simulink model "BCS_v1_2018a"  (R2018a)
settings: Solver=ode5  StartTime=0.0  StopTime=inf  FixedStep=sampletime  RelTol=1e-3  EnableMultiTasking=on
values from neighbouring files (symbols this model uses):
  extension_lower = 0    [Ignition.m]
  extension_upper = 1800    [Ignition.m]
  kd4 = 1e-2    (= 0.01)    [Ignition.m]
  kq1 = 0.1    [Ignition.m]
  kq2 = 0.1    [Ignition.m]
  kq3 = 0.1    [Ignition.m]
  lift_lower = 0    [Ignition.m]
  lift_upper = 75    [Ignition.m]
  Max_1 = 5    [Ignition.m]
  Max_2 = 5    [Ignition.m]
  Max_3 = 5    [Ignition.m]
  Max_4 = 10    [Ignition.m]
  Max_rot = 5    [Ignition.m]
  Max_x = 0.1    [Ignition.m]
  Max_y = 0.1    [Ignition.m]
  rotation_lower = -140    [Ignition.m]
  rotation_upper = 140    [Ignition.m]
  tilt_lower = -175    [Ignition.m]
  tilt_upper = -10    [Ignition.m]
libraries: simulink x4, xpcrtudplib x2, etargetslib x1, xpcutilitieslib x1
settings Model: Creator=leduc  LastModifiedBy=led
settings SolverCC: ConcurrentTasks=on  AutoInsertRateTranBlk=on
settings DataIOCC: SaveFormat=StructureWithTime
settings OptimizationCC: BlockReduction=off  OptimizeBlockIOStorage=off  BufferReuse=off  GlobalBufferReuse=off  ExpressionFolding=off  LocalBlockOutputs=off  OptimizeDataStoreBuffers=off  BusAssignmentInplaceUpdate=off
settings DebuggingCC: LibraryContextMissingDiagnostic=warning
settings HardwareCC: ProdBitPerPointer=32  ProdBitPerSizeT=32  ProdBitPerPtrDiffT=32  ProdLargestAtomicFloat=None  ProdWordSize=32  ProdLongLongMode=on  ProdHWDeviceType=Generic->32-bit x86 compatible
settings SFSimCC: SimUseLocalCustomCode=on
settings RTWCC: SystemTargetFile=slrt.tlc  TemplateMakefile=slrt_default_tmf  Description=Simulink Real-Time  RTWUseLocalCustomCode=on  CodeExecutionProfiling=on  RTWCompilerOptimization=on
settings SimulinkRealTimeCC: RL32LogTETModifier=off  xPCisDownloadable=off  xPCConcurrentTasks=on

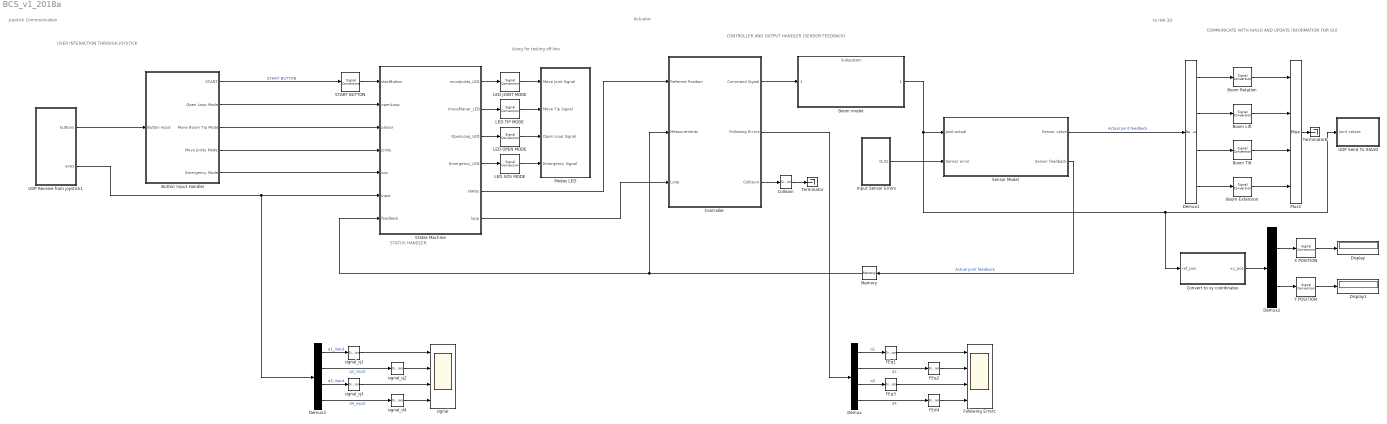
== system BCS_v1_2018a ==
  note: Using for testing off-line
  note: USER INTERACTION THROUGH JOYSTICK
  note: Joystick Communication
  note: COMMUNICATE WITH IHA3D AND
      | UPDATE INFORMATION FOR GUI
  note: CONTROLLER AND OUTPUT HANDLER (SENSOR FEEDBACK)
  note: STATUS HANDLER
  note: to IHA 3D
  note: Actuator
  Boom Extension : SignalConversion  OverrideOpt=off
  Boom Lift : SignalConversion  OverrideOpt=off
  Boom Rotation : SignalConversion  OverrideOpt=off
  Boom Tilt : SignalConversion  OverrideOpt=off
  Boom model : ModelReference  ModelNameDialog=Subsystem.slxp  ModelReferenceVersion=1.514  CopyOfModelProtected=on
  Button Input Handler : Subsystem
  Collision : SignalConversion  OverrideOpt=off
  Controller : Subsystem
  Convert to xy coordinates : MATLAB Function  TreatAsAtomicUnit=on
  Demux : Demux
  Demux1 : Demux
  Demux2 : Demux  Outputs=2
  Demux3 : Demux
  Display : Display
  Display1 : Display
  FEd4 : SignalConversion  OverrideOpt=off
  FEq1 : SignalConversion  OverrideOpt=off
  FEq2 : SignalConversion  OverrideOpt=off
  FEq3 : SignalConversion  OverrideOpt=off
  Following Errors : Scope  NumInputPorts=4
  Input Sensor Errors : Subsystem
  LED JOINT MODE : SignalConversion  OverrideOpt=off
  LED OPEN MODE : SignalConversion  OverrideOpt=off
  LED SOS MODE : SignalConversion  OverrideOpt=off
  LED TIP MODE : SignalConversion  OverrideOpt=off
  Memory : Memory
  Modes LED : Subsystem
  Mux1 : Mux
  START BUTTON : SignalConversion  OverrideOpt=off
  Sensor Model : Subsystem
  States Machine : Stateflow chart  TreatAsAtomicUnit=on
  Terminator : Terminator
  Terminator6 : Terminator
  UDP Receive from joystick1 : Subsystem
  UDP Send To IHA3D : Subsystem
  X POSITION : SignalConversion  OverrideOpt=off
  Y POSITION : SignalConversion  OverrideOpt=off
  signal : Scope  NumInputPorts=4
  signal_d4 : SignalConversion  OverrideOpt=off
  signal_q1 : SignalConversion  OverrideOpt=off
  signal_q2 : SignalConversion  OverrideOpt=off
  signal_q3 : SignalConversion  OverrideOpt=off
  wires:
  Input Sensor Errors/1(Out1) -> Sensor Model/2(Sensor error)
  Controller/1(Command Signal) -> Boom model/1
  States Machine/6(loop) -> Controller/3(Loop)
  States Machine/5(states) -> Controller/1(Referent Position)
  Boom model/1 -> Convert to xy coordinates/1(ref_pos), UDP Send To IHA3D/1(joint values), Sensor Model/1(Joint actual)
  UDP Receive from joystick1/2(axes) -> Demux3/1, States Machine/6(input)
  Memory/1 -> States Machine/7(feedback), Controller/2(Measurements)
  UDP Receive from joystick1/1(buttons) -> Button Input Handler/1(Button Input)
  START BUTTON/1 -> States Machine/1(startButton)
  States Machine/2(movePlanar_LED) -> LED TIP MODE/1
  States Machine/3(OpenLoop_LED) -> LED OPEN MODE/1
  States Machine/4(Emergency_LED) -> LED SOS MODE/1
  Sensor Model/2(Sensor feedback) -> Memory/1  "Actual Joint feedback"
  States Machine/1(moveJoints_LED) -> LED JOINT MODE/1
  LED TIP MODE/1 -> Modes LED/2(Move Tip Signal)
  LED OPEN MODE/1 -> Modes LED/3(Open Loop Signal)
  LED SOS MODE/1 -> Modes LED/4(Emergency Signal)
  FEd4/1 -> Following Errors/4
  Demux/2 -> FEq2/1  "q2"
  FEq3/1 -> Following Errors/3
  FEq2/1 -> Following Errors/2
  Demux/1 -> FEq1/1  "q1"
  Demux/4 -> FEd4/1  "d4"
  Demux/3 -> FEq3/1  "q3"
  Controller/2(Following Errors) -> Demux/1
  FEq1/1 -> Following Errors/1
  Demux1/1 -> Boom Rotation/1
  Boom Lift/1 -> Mux1/2
  Boom Rotation/1 -> Mux1/1
  Demux1/2 -> Boom Lift/1
  Demux1/3 -> Boom Tilt/1
  Boom Tilt/1 -> Mux1/3
  Demux1/4 -> Boom Extension/1
  Convert to xy coordinates/1(xy_pos) -> Demux2/1
  Y POSITION/1 -> Display1/1
  Boom Extension/1 -> Mux1/4
  Demux2/1 -> X POSITION/1
  Demux2/2 -> Y POSITION/1
  X POSITION/1 -> Display/1
  Sensor Model/1(Sensor value) -> Demux1/1  "Actual Joint feedback"
  LED JOINT MODE/1 -> Modes LED/1(Move Joint Signal)
  Button Input Handler/3(Move Boom Tip Mode) -> States Machine/3(planar)
  Button Input Handler/5(Emergency Mode) -> States Machine/5(sos)
  Button Input Handler/4(Move Joints Mode) -> States Machine/4(joints)
  Button Input Handler/1(START) -> START BUTTON/1  "START BUTTON"
  Mux1/1 -> Terminator6/1
  Button Input Handler/2(Open Loop Mode) -> States Machine/2(openLoop)
  signal_q1/1 -> signal/1
  Demux3/3 -> signal_q3/1  "q3_input"
  Demux3/4 -> signal_d4/1  "d4_input"
  Demux3/1 -> signal_q1/1  "q1_input"
  signal_q2/1 -> signal/2
  signal_q3/1 -> signal/3
  Demux3/2 -> signal_q2/1  "q2_input"
  signal_d4/1 -> signal/4
  Collision/1 -> Terminator/1
  Controller/3(Collision) -> Collision/1

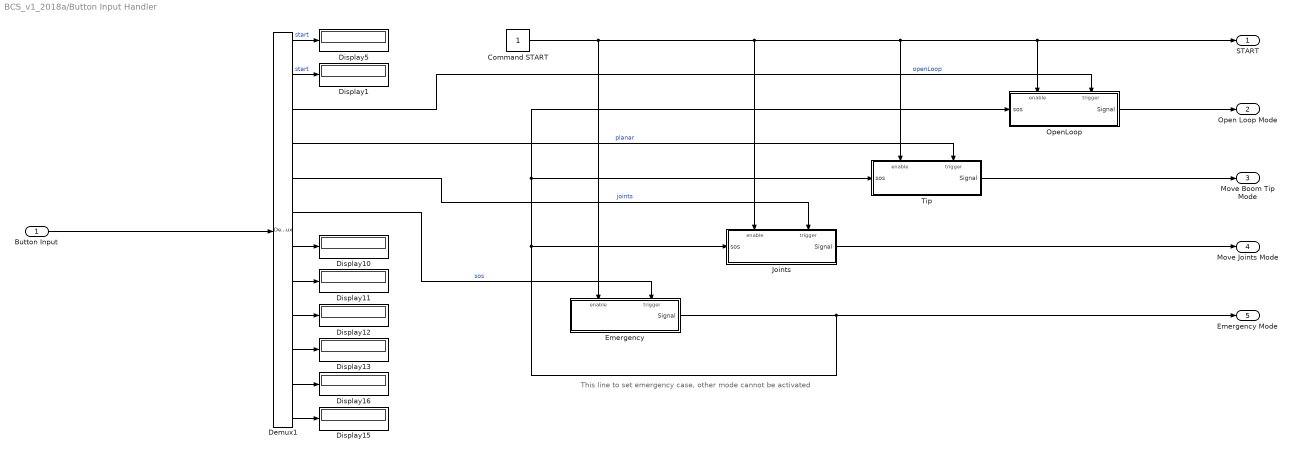
== system BCS_v1_2018a/Button Input Handler ==
  note: This line to set emergency case, other mode cannot be activated
  Button Input : Inport
  Command START : Constant
  Demux1 : Demux  Outputs=12
  Display{1,5,10..13,15..16} (8 alike) : Display
  Emergency : Subsystem
  Joints : Subsystem
  OpenLoop : Subsystem
  Tip : Subsystem
  START : Outport
  Open Loop Mode : Outport  Port=2
  Move Boom Tip Mode : Outport  Port=3
  Move Joints Mode : Outport  Port=4
  Emergency Mode : Outport  Port=5
  wires:
  Demux1/11 -> Display16/1
  Demux1/8 -> Display11/1
  Demux1/6 -> Emergency/Trigger  "sos"
  Demux1/3 -> OpenLoop/Trigger  "openLoop"
  Demux1/12 -> Display15/1
  Demux1/9 -> Display12/1
  Demux1/10 -> Display13/1
  Demux1/7 -> Display10/1
  Demux1/4 -> Tip/Trigger  "planar"
  Demux1/5 -> Joints/Trigger  "joints"
  Button Input/1 -> Demux1/1
  Demux1/2 -> Display1/1  "start"
  Demux1/1 -> Display5/1  "start"
  OpenLoop/1(Signal) -> Open Loop Mode/1
  Tip/1(Signal) -> Move Boom Tip Mode/1
  Joints/1(Signal) -> Move Joints Mode/1
  Emergency/1(Signal) -> Joints/1(sos), Tip/1(sos), OpenLoop/1(sos), Emergency Mode/1
  Command START/1 -> Emergency/Enable, Joints/Enable, OpenLoop/Enable, START/1, Tip/Enable

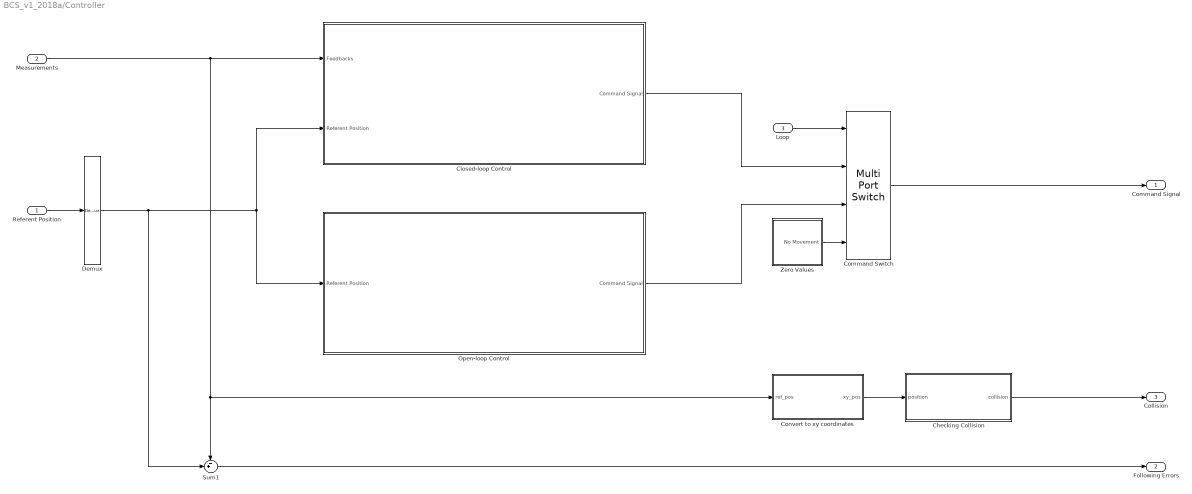
== system BCS_v1_2018a/Controller ==
  Referent Position : Inport
  Measurements : Inport  Port=2
  Loop : Inport  Port=3
  Checking Collision : MATLAB Function  TreatAsAtomicUnit=on
  Closed-loop Control : Subsystem
  Command Switch : MultiPortSwitch  DataPortOrder=Specify indices  Inputs=2  DataPortIndices={1,2}  DataPortForDefault=Additional data port  DiagnosticForDefault=None
  Convert to xy coordinates : MATLAB Function  TreatAsAtomicUnit=on
  Demux : Demux  Outputs=1
  Open-loop Control : Subsystem
  Sum1 : Sum  Inputs=-+|
  Zero Values : Subsystem
  Command Signal : Outport
  Following Errors : Outport  Port=2
  Collision : Outport  Port=3
  wires:
  Open-loop Control/1(Command Signal) -> Command Switch/3
  Referent Position/1 -> Demux/1
  Demux/1 -> Sum1/2, Open-loop Control/1(Referent Position), Closed-loop Control/2(Referent Position)
  Loop/1 -> Command Switch/1
  Closed-loop Control/1(Command Signal) -> Command Switch/2
  Measurements/1 -> Closed-loop Control/1(Feedbacks), Convert to xy coordinates/1(ref_pos), Sum1/1
  Sum1/1 -> Following Errors/1
  Zero Values/1(No Movement) -> Command Switch/4
  Checking Collision/1(collision) -> Collision/1
  Command Switch/1 -> Command Signal/1
  Convert to xy coordinates/1(xy_pos) -> Checking Collision/1(position)

== system BCS_v1_2018a/Input Sensor Errors ==
  Mux : Mux
  Step{,1..3} (4 alike) : Step  Time=3  After=0.1  SampleTime=0
  Out1 : Outport
  wires:
  Step2/1 -> Mux/3
  Step/1 -> Mux/1
  Step3/1 -> Mux/4
  Step1/1 -> Mux/2
  Mux/1 -> Out1/1

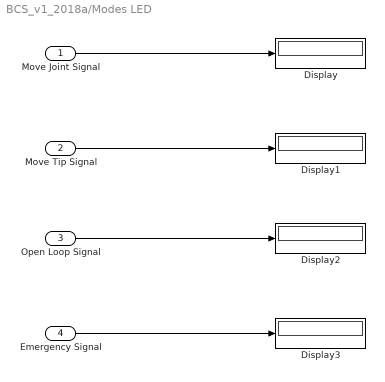
== system BCS_v1_2018a/Modes LED ==
  Move Joint Signal : Inport
  Move Tip Signal : Inport  Port=2
  Open Loop Signal : Inport  Port=3
  Emergency Signal : Inport  Port=4
  Display{,1..3} (4 alike) : Display
  wires:
  Move Joint Signal/1 -> Display/1
  Move Tip Signal/1 -> Display1/1
  Emergency Signal/1 -> Display3/1
  Open Loop Signal/1 -> Display2/1

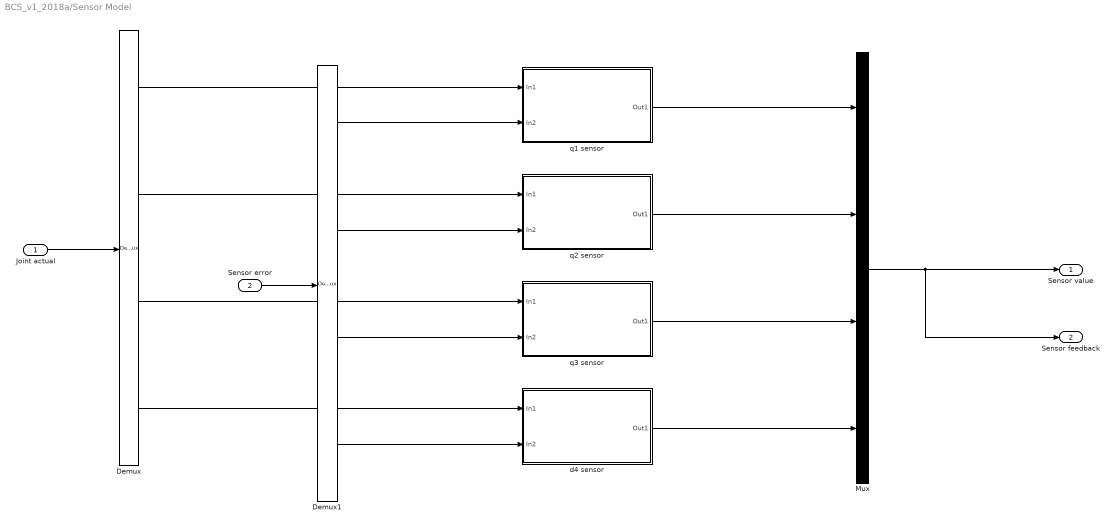
== system BCS_v1_2018a/Sensor Model ==
  Joint actual : Inport
  Sensor error : Inport  Port=2
  Demux : Demux
  Demux1 : Demux
  Mux : Mux
  d4 sensor : Subsystem
  q1 sensor : Subsystem
  q2 sensor : Subsystem
  q3 sensor : Subsystem
  Sensor value : Outport
  Sensor feedback : Outport  Port=2
  wires:
  d4 sensor/1(Out1) -> Mux/4
  q3 sensor/1(Out1) -> Mux/3
  q2 sensor/1(Out1) -> Mux/2
  q1 sensor/1(Out1) -> Mux/1
  Mux/1 -> Sensor feedback/1, Sensor value/1
  Demux/1 -> q1 sensor/1(In1)
  Demux/2 -> q2 sensor/1(In1)
  Demux/4 -> d4 sensor/1(In1)
  Demux/3 -> q3 sensor/1(In1)
  Demux1/1 -> q1 sensor/2(In2)
  Demux1/2 -> q2 sensor/2(In2)
  Demux1/3 -> q3 sensor/2(In2)
  Demux1/4 -> d4 sensor/2(In2)
  Sensor error/1 -> Demux1/1
  Joint actual/1 -> Demux/1

== system BCS_v1_2018a/UDP Receive from joystick1 ==
  Byte Unpack : etargetslib/Byte Unpack  dimensions={4,12}  datatypes={'double','uint8'}  byteAlign=1
  Terminator : Terminator
  UDP Receive : xpcrtudplib/UDP Receive  ipAddressVal=Use host-target connection  localPort=55550  rcvWidth=44  rcvFmAny=off  fmAddress=192.168.10.1  rcvMulticast=off  multicastAddress=[]  maxUDPQueue=8  sampleTime=sampletime
      settings: SourceProductName=Simulink Real-Time
  buttons : Outport
  axes : Outport  Port=2
  wires:
  UDP Receive/2 -> Terminator/1
  UDP Receive/1 -> Byte Unpack/1
  Byte Unpack/1 -> axes/1  "axes"
  Byte Unpack/2 -> buttons/1  "buttons"

== system BCS_v1_2018a/UDP Send To IHA3D ==
  note: Frequency rate:
      | How often UDP message is sent
      | 1: every sample time
      | 2: every second sample time
      | 3: every third sample time
      | 4: etc....
  joint values : Inport
  Enabled Subsystem : Subsystem  TreatAsAtomicUnit=on
  Frequency rate : Constant
  Subsystem : Subsystem
  gain : Gain  Gain=[1 1 1 1]
  wires:
  Subsystem/1(enable) -> Enabled Subsystem/Enable
  Frequency rate/1 -> Subsystem/1(freq)
  joint values/1 -> gain/1
  gain/1 -> Enabled Subsystem/1(q)

== system BCS_v1_2018a/Button Input Handler/Emergency ==
  Enable : EnablePort
  Trigger : TriggerPort  VariantControl=Variant  PortDimensions=1
  Convert_SoS : MATLAB Function  TreatAsAtomicUnit=on
  Signal : Outport
  wires:
  Convert_SoS/1(y) -> Signal/1

== system BCS_v1_2018a/Button Input Handler/Joints ==
  sos : Inport
  Enable : EnablePort
  Trigger : TriggerPort  VariantControl=Variant  PortDimensions=1
  Convert : MATLAB Function  TreatAsAtomicUnit=on
  Signal : Outport
  wires:
  sos/1 -> Convert/1(u)
  Convert/1(y) -> Signal/1

== system BCS_v1_2018a/Button Input Handler/OpenLoop ==
  sos : Inport
  Enable : EnablePort
  Trigger : TriggerPort  VariantControl=Variant  PortDimensions=1
  Convert : MATLAB Function  TreatAsAtomicUnit=on
  Signal : Outport
  wires:
  sos/1 -> Convert/1(u)
  Convert/1(y) -> Signal/1

== system BCS_v1_2018a/Button Input Handler/Tip ==
  sos : Inport
  Enable : EnablePort
  Trigger : TriggerPort  VariantControl=Variant  PortDimensions=1
  Convert : MATLAB Function  TreatAsAtomicUnit=on
  Signal : Outport
  wires:
  sos/1 -> Convert/1(u)
  Convert/1(y) -> Signal/1

== system BCS_v1_2018a/Controller/Closed-loop Control ==
  Feedbacks : Inport
  Referent Position : Inport  Port=2
  P Control : Subsystem
  Sum1 : Sum  Inputs=-+|
  Command Signal : Outport
  wires:
  Referent Position/1 -> Sum1/2
  Feedbacks/1 -> Sum1/1
  Sum1/1 -> P Control/1(In1)
  P Control/1(Out1) -> Command Signal/1

== system BCS_v1_2018a/Controller/Open-loop Control ==
  Referent Position : Inport
  P Control : Subsystem
  Command Signal : Outport
  wires:
  Referent Position/1 -> P Control/1(In1)  "DIRECTLY COMMAND FROM JOYSTICK"
  P Control/1(Out1) -> Command Signal/1

== system BCS_v1_2018a/Controller/Zero Values ==
  Constant{,1..3} (4 alike) : Constant  Value=0
  Mux : Mux
  No Movement : Outport
  wires:
  Constant3/1 -> Mux/4
  Constant1/1 -> Mux/2
  Mux/1 -> No Movement/1
  Constant/1 -> Mux/1
  Constant2/1 -> Mux/3

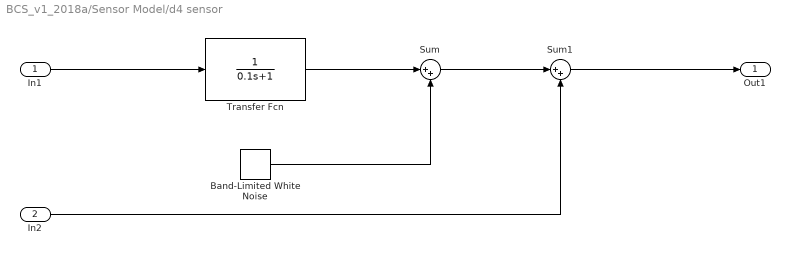
== system BCS_v1_2018a/Sensor Model/d4 sensor ==
  In1 : Inport
  In2 : Inport  Port=2
  Band-Limited White Noise : simulink/Sources/Band-Limited White Noise  Cov=[0.00001]  Ts=sampletime  seed=[23341]
  Sum : Sum  Inputs=|++
  Sum1 : Sum  Inputs=|++
  Transfer Fcn : TransferFcn  Denominator=[0.1 1]
  Out1 : Outport
  wires:
  In2/1 -> Sum1/2
  Band-Limited White Noise/1 -> Sum/2
  Sum1/1 -> Out1/1
  Sum/1 -> Sum1/1
  Transfer Fcn/1 -> Sum/1
  In1/1 -> Transfer Fcn/1

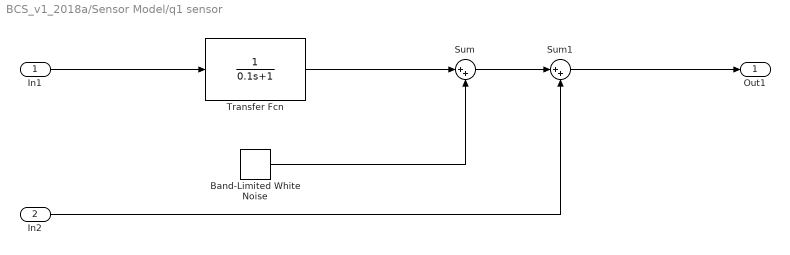
== system BCS_v1_2018a/Sensor Model/q1 sensor ==
  In1 : Inport
  In2 : Inport  Port=2
  Band-Limited White Noise : simulink/Sources/Band-Limited White Noise  Cov=[0.00001]  Ts=sampletime  seed=[23341]
  Sum : Sum  Inputs=|++
  Sum1 : Sum  Inputs=|++
  Transfer Fcn : TransferFcn  Denominator=[0.1 1]
  Out1 : Outport
  wires:
  Sum/1 -> Sum1/1
  Sum1/1 -> Out1/1
  Band-Limited White Noise/1 -> Sum/2
  In2/1 -> Sum1/2
  Transfer Fcn/1 -> Sum/1
  In1/1 -> Transfer Fcn/1

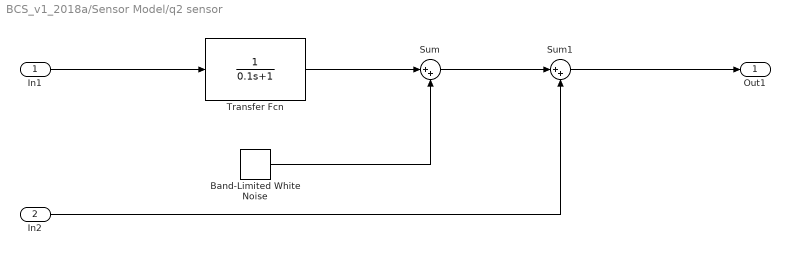
== system BCS_v1_2018a/Sensor Model/q2 sensor ==
  In1 : Inport
  In2 : Inport  Port=2
  Band-Limited White Noise : simulink/Sources/Band-Limited White Noise  Cov=[0.00001]  Ts=sampletime  seed=[23341]
  Sum : Sum  Inputs=|++
  Sum1 : Sum  Inputs=|++
  Transfer Fcn : TransferFcn  Denominator=[0.1 1]
  Out1 : Outport
  wires:
  In2/1 -> Sum1/2
  Band-Limited White Noise/1 -> Sum/2
  Sum1/1 -> Out1/1
  Sum/1 -> Sum1/1
  Transfer Fcn/1 -> Sum/1
  In1/1 -> Transfer Fcn/1

== system BCS_v1_2018a/Sensor Model/q3 sensor ==
  In1 : Inport
  In2 : Inport  Port=2
  Band-Limited White Noise : simulink/Sources/Band-Limited White Noise  Cov=[0.00001]  Ts=sampletime  seed=[23341]
  Sum : Sum  Inputs=|++
  Sum1 : Sum  Inputs=|++
  Transfer Fcn : TransferFcn  Denominator=[0.1 1]
  Out1 : Outport
  wires:
  In1/1 -> Transfer Fcn/1
  Transfer Fcn/1 -> Sum/1
  Sum/1 -> Sum1/1
  Sum1/1 -> Out1/1
  Band-Limited White Noise/1 -> Sum/2
  In2/1 -> Sum1/2

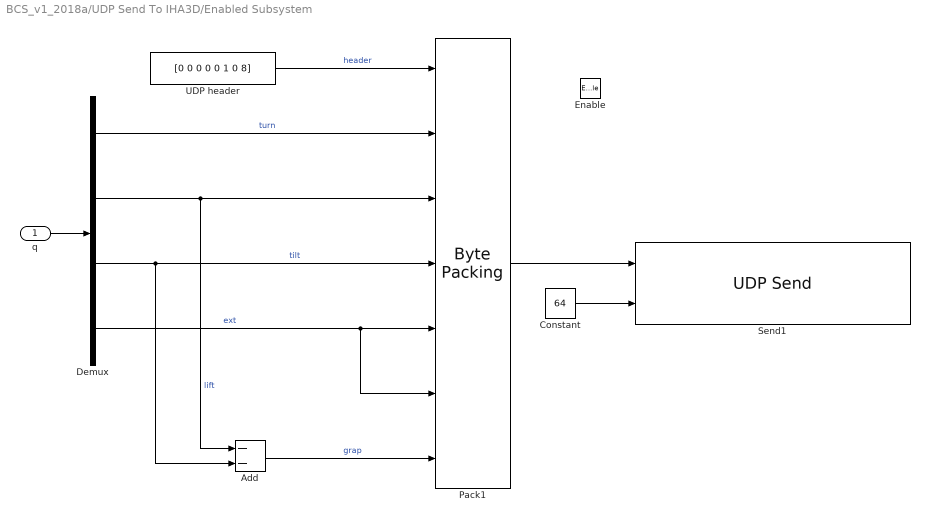
== system BCS_v1_2018a/UDP Send To IHA3D/Enabled Subsystem ==
  q : Inport
  Enable : EnablePort
  Add : Sum  Inputs=--
  Constant : Constant  Value=64
  Demux : Demux
  Pack1 : xpcutilitieslib/Byte Packing   MaskPackedDataType=uint8  MaskUnpackedDataTypes={'uint8','double','double','double','double','double','double'}  MaskAlignment=1
  Send1 : xpcrtudplib/UDP Send  ipAddressVal=Use host-target connection  localPort=5555  toAddress=192.168.10.1  toPort=7755  sampleTime=sampletime
      settings: SourceProductName=Simulink Real-Time  SourceProductBaseCode=XP
  UDP header : Constant  Value=[0 0 0 0 0 1 0 8]  OutDataTypeStr=uint8
  wires:
  UDP header/1 -> Pack1/1  "header"
  q/1 -> Demux/1
  Demux/2 -> Pack1/3, Add/1  "lift"
  Demux/3 -> Pack1/4, Add/2  "tilt"
  Demux/4 -> Pack1/6, Pack1/5  "ext"
  Add/1 -> Pack1/7  "grap"
  Demux/1 -> Pack1/2  "turn"
  Pack1/1 -> Send1/1
  Constant/1 -> Send1/2

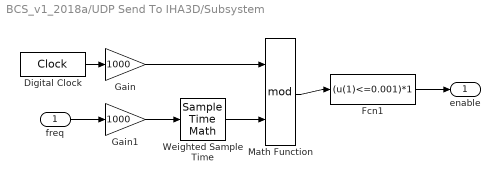
== system BCS_v1_2018a/UDP Send To IHA3D/Subsystem ==
  freq : Inport
  Digital Clock : DigitalClock  SampleTime=sampletime
  Fcn1 : Fcn  Expr=(u(1)<=0.001)*1
  Gain : Gain  Gain=1000
  Gain1 : Gain  Gain=1000  SampleTime=sampletime
  Math Function : Math  Operator=mod  SaturateOnIntegerOverflow=on
  Weighted Sample Time : SampleTimeMath  TsampMathOp=*
  enable : Outport
  wires:
  Weighted Sample Time/1 -> Math Function/2
  freq/1 -> Gain1/1
  Math Function/1 -> Fcn1/1
  Gain/1 -> Math Function/1
  Gain1/1 -> Weighted Sample Time/1
  Fcn1/1 -> enable/1
  Digital Clock/1 -> Gain/1

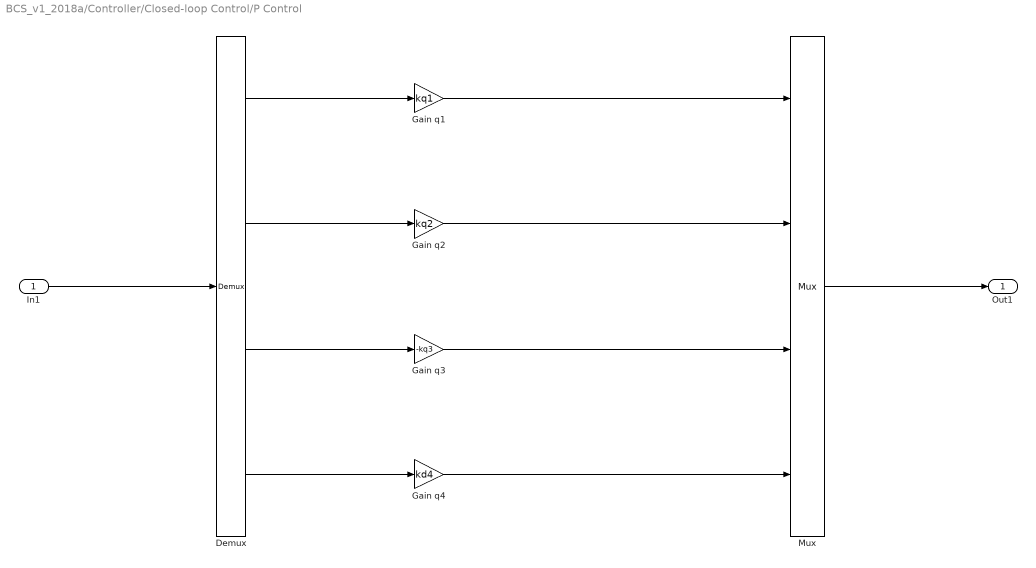
== system BCS_v1_2018a/Controller/Closed-loop Control/P Control ==
  In1 : Inport
  Demux : Demux
  Gain q1 : Gain  Gain=kq1
  Gain q2 : Gain  Gain=kq2
  Gain q3 : Gain  Gain=-kq3
  Gain q4 : Gain  Gain=kd4
  Mux : Mux
  Out1 : Outport
  wires:
  Mux/1 -> Out1/1
  In1/1 -> Demux/1
  Demux/1 -> Gain q1/1
  Gain q1/1 -> Mux/1
  Demux/2 -> Gain q2/1
  Demux/3 -> Gain q3/1
  Demux/4 -> Gain q4/1
  Gain q2/1 -> Mux/2
  Gain q3/1 -> Mux/3
  Gain q4/1 -> Mux/4

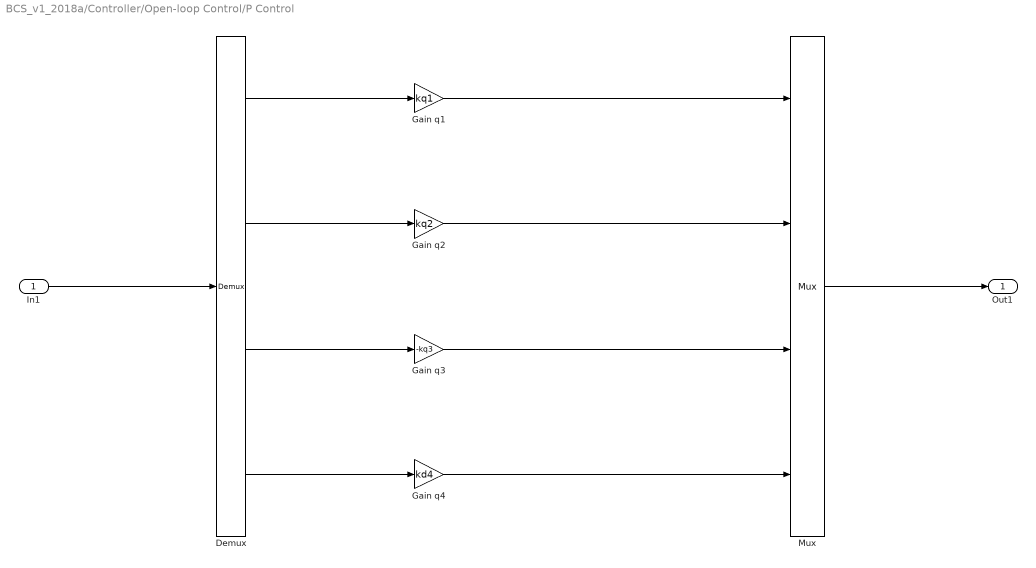
== system BCS_v1_2018a/Controller/Open-loop Control/P Control ==
  In1 : Inport
  Demux : Demux
  Gain q1 : Gain  Gain=kq1
  Gain q2 : Gain  Gain=kq2
  Gain q3 : Gain  Gain=-kq3
  Gain q4 : Gain  Gain=kd4
  Mux : Mux
  Out1 : Outport
  wires:
  Mux/1 -> Out1/1
  In1/1 -> Demux/1
  Demux/1 -> Gain q1/1
  Gain q1/1 -> Mux/1
  Demux/2 -> Gain q2/1
  Demux/3 -> Gain q3/1
  Demux/4 -> Gain q4/1
  Gain q2/1 -> Mux/2
  Gain q3/1 -> Mux/3
  Gain q4/1 -> Mux/4

== stateflow chart BCS_v1_2018a/States Machine ==
  settings: executeAtInitialization=1
  state Idle
    entry:
    disp('Idle entry')
    during:
    disp('Waiting entry')
    exit:
    disp('Idle exit')
  state Operation
    entry:
    disp('Operation entry')
    during:
    disp('Operation during')
    Max_vel = [Max_1; Max_2; Max_3;Max_4];
    Max_xy = [Max_x; Max_y; Max_rot];
    Limits = [[rotation_lower,rotation_upper];...
    [lift_lower,lift_upper];...
    [tilt_lower,tilt_upper];...
    [extension_lower,extension_upper]];
    exit:
    disp('Operation exit')
    state Move_Joints
      entry:
      disp('Move Joints')
      Recovery = 1
      moveJoints_LED = 1;loop = 1; % Chose Closed-loop control
      initial_position = feedback
      during:
      disp('Moving Joints')
      states_raw = Move_joints(feedback, input,...
      Max_vel, initial_position);
      states = checkFeedback(states_raw, Limits);
      loop = FK(states);
      exit:
      disp('Done')
      moveJoints_LED = 0;
    state Move_Boom_Tip
      entry:
      disp('Move Boom Tip')
      Recovery = 2
      movePlanar_LED = 1;loop = 1;
      initial_position = feedback;
      during:
      disp('Moving Boom Tip')
      qvel = IK_vel(feedback, input, Max_xy);
      states_raw = Move_Tip(feedback, qvel,...
      initial_position);
      states = checkFeedback(states_raw, Limits);
      loop = FK(states);
      exit:
      disp('Done')
      movePlanar_LED = 0;
    state waiting
      entry:
      Recovery = 0;
      disp('change mode')
      loop = 0;
      during: disp('changing')
      exit: disp('changed')
    state Emergency
      entry:
      disp('Emergency')
      loop = 0;
      Emergency_LED = 1;
      during:
      disp('Stop everything')
      exit:
      disp('Return normal')
      Emergency_LED = 0;
    state Move_Open_Loop
      entry:
      Recovery = 3
      OpenLoop_LED = 1; loop = 2;
      disp('Change to Open Loop')
      during:
      disp('Manual Control')
      feedback_ = checkFb_openloop(feedback, Limits, input);
      states = feedback_ .* Max_vel;
      exit:
      disp('Done')
      OpenLoop_LED = 0;
    Move_Joints -> Emergency [order 2] : [sos == 1]
    Emergency -> Move_Joints [order 4] : [sos == 0 && Recovery == 1]
    waiting -> Move_Joints [order 1] : [joints == 1]
    Move_Joints -> waiting [order 1] : [joints == 0]
    Emergency -> Move_Boom_Tip [order 3] : [sos == 0 && Recovery == 2]
    Move_Boom_Tip -> Emergency [order 2] : [sos == 1]
    (default) -> waiting
    waiting -> Move_Boom_Tip [order 3] : [planar == 1]
    Move_Boom_Tip -> waiting [order 1] : [planar == 0]
    Emergency -> waiting [order 1] : [sos == 0 && Recovery == 0]
    waiting -> Emergency [order 4] : [sos == 1]
    waiting -> Move_Open_Loop [order 2] : [openLoop == 1]
    Move_Open_Loop -> waiting [order 1] : [openLoop == 0]
    Move_Open_Loop -> Emergency [order 2] : [sos == 1]
    Emergency -> Move_Open_Loop [order 2] : [sos == 0 && Recovery == 3]
  (default) -> Idle
  Idle -> Operation : [startButton == 1]/{disp('ignition')}
  Operation -> Idle : [startButton == 0]/{disp('stop')}
  data: measurements function_input; jst_input function_input; q_vel function_output; Maxi_xy function_input; loop_control function_output; ref_pos function_input; measurements function_input; jst_input function_input; ref_position function_output; Maxi_vel function_input; initial_pos function_input; measurements function_input; vel_input function_input; ref_position function_output; initial_pos function_input; checked_feedback function_output; measurements function_input; LimitsJoints function_input; checked_input function_output; measurements function_input; LimitsJoints function_input; jst_input function_input; startButton input; openLoop input; planar input; joints input; moveJoints_LED output; movePlanar_LED output; OpenLoop_LED output; sos input; Emergency_LED output; input input; feedback input; states output; sampletime parameter; loop output; Max_vel local; Limits local; qvel local; xy_ref local; initial_position local; feedback_ local; Recovery local; rotation_lower parameter; lift_lower parameter; extension_lower parameter; extension_upper parameter; tilt_lower parameter; tilt_upper parameter; lift_upper parameter; rotation_upper parameter; Max_1 parameter; Max_2 parameter; Max_3 parameter; Max_4 parameter; states_raw local; Max_x parameter; Max_y parameter; Max_rot parameter; Max_xy local
  function q_vel = IK_vel(measurements, jst_input, Maxi_xy):
    | function q_vel = IK_vel(measurements, jst_input, Maxi_xy)
    | % This function transforms desired coordinate velocities to desired joint
    | % velocities in such a way that the joints move as little as possible. To
    | % do this, the function needs to also know the current pose (joint
    | % positions) of the manipulator.
    | %
    | % Notice that the output is a set of desired joint velocities, not
    | % absolute joint positions. If you know the discrete time step you are
    | % using, you can integrate those velocities into a change of position.
    | %
    | % Likewise, the inputs xvel & yvel are desired coordinate velocities, not
    | % desired absolute coordinate positions. If you want to explicitly control
    | % coordinate positions, you can calculate the time derivative of your
    | % desired coordinate positions to get the desired velocities.
    | %
    | % The first joint angle, q1, has no effect on the kinematics, so it is not
    | % a part of this function.
    | % Inputs:
    | %   measurements        - feedback data of joints position
    | %   jst_input           - joystick input signals
    | %   Maxi_xy             - Desired Maximum velocities in planar mode
    | %
    | %  Outputs:
    | %   qvel                - Joints velocities
    | %
    | % Locals: 
    | %   q2,q3,d4            - Current joint position references
    | %                         e.g. from last iteration [deg,m]
    | %   xvel,yvel           - Desired coordinate velocities [m/s]
    | %
    | %   q2vel,q3vel,d4vel   - Desired joint velocities [deg/s,m/s]
    | %
    | 
    | % Modify input joint position
    | q2 = measurements(2);
    | q3 = measurements(3);
    | d4 = measurements(4)/1000;
    | 
    | % Modify input xy velocities 
    | xvel = Maxi_xy(1) * jst_input(1);
    | yvel = Maxi_xy(2) * jst_input(2);
    | q1vel = Maxi_xy(3) * jst_input(3); 
    | 
    | % Unit conversion to radians and meters
    | deg_to_rad = pi/180;
    | rad_to_deg = 180/pi;
    | q2 = q2*deg_to_rad;
    | q3 = q3*deg_to_rad;
    | 
    | % Calculate the [3*2] Jacobian pseudoinverse
    | t1 = sin(q2);
    | t2 = q3 + pi / 0.2e1;
    | t3 = cos(t2);
    | t4 = cos(q2);
    | t2 = sin(t2);
    | t5 = -t1 * t2 + t3 * t4;
    | t6 = d4 + 0.213e1;
    | t7 = t4 * t2;
    | t8 = t1 * t3;
    | t9 = t7 + t8;
    | t10 = 0.350440540000000000e1;
    | t11 = t9 * 0.376348799999999983e0;
    | t12 = t5 * t6;
    | t13 = -t1 * t10 - t11 + t12;
    | t14 = t1 ^ 2;
    | t15 = t14 ^ 2;
    | t16 = t4 ^ 2;
    | t17 = t16 ^ 2;
    | t18 = t3 ^ 2;
    | t19 = t18 ^ 2;
    | t20 = t7 * t1;
    | t21 = t1 * t18 * t4;
    | t22 = d4 * (t2 * (t3 * (-t16 + t14) + t20) - t21);
    | t23 = t4 * t9;
    | t24 = t2 ^ 2;
    | t25 = t24 ^ 2;
    | t26 = t14 * t18 + t16 * t24;
    | t27 = d4 ^ 2;
    | t28 = -t16 + t14;
    | t29 = t3 * t28;
    | t30 = t2 * (t20 + t29) - t21;
    | t31 = t14 * t24 + t16 * t18;
    | t32 = 0.1492876700e2;
    | t33 = 0.7008810800e1;
    | t34 = 0.2637757534e1;
    | t35 = 0.1283276839e1;
    | t36 = 0.8520000000e1;
    | t37 = 0.9073800000e1;
    | t38 = (0.4e1 * d4 + 0.1704000000e2) * d4;
    | t39 = 0.1505395200e1 * t22;
    | t40 = 0.3206491776e1 * t30;
    | t8 = d4 * t23 * t33 + d4 * t26 * t36 + t34 * t4 * t5 + t23 * t32 + 0.2e1 * t27 * t26 + t26 * t37 + t31 * t35 + t4 * (0.1228085721e2 * t4 + t8 * t2 * (t38 + 0.1558104632e2)) - t39 - t40;
    | t23 = t18 + t24;
    | t23 = t2 * (t15 * t23 + t17 * t23);
    | t41 = t18 + t24;
    | t42 = t14 * t16;
    | t43 = t42 * t2;
    | t44 = t17 + t15;
    | t45 = t3 * t2;
    | t46 = t42 * t24;
    | t47 = t42 * t19;
    | t48 = t24 * (t18 * (t17 + t15) + t46) + t47;
    | t49 = t18 * t44;
    | t50 = t19 + t25;
    | t50 = t15 * t50 + t17 * t50;
    | t19 = t19 + t25;
    | t25 = 0.9073800003e1;
    | t51 = 0.1814760000e2;
    | t15 = d4 * t23 * t33 + 0.1401762160e2 * t43 * d4 * t41 - 0.9243771744e1 * t45 * d4 * t44 + 0.2985753400e2 * t43 * t41 + 0.5231645170e2 * t49 * d4 - 0.1968923382e2 * t45 * t44 + 0.1228085721e2 * t49 * t27 + t51 * (t24 * (t46 + t49) + t47) + 0.8519999996e1 * d4 * t50 + t23 * t32 + t25 * (t15 * t19 + t17 * t19) + 0.1402029841e2 * t24 * t44 + 0.5571702104e2 * t49 + 0.1704000000e2 * d4 * t48 + 0.4e1 * t27 * t48 + 0.2e1 * t27 * t50 + t42 * (t3 * (t2 * (-0.1848754340e2 * d4 - 0.3937846770e2) + t3 * (((0.8e1 * t24 + 0.2456171442e2) * d4 + 0.3408000000e2 * t24 + 0.1046329034e3) * d4 + 0.3629520000e2 * t24 + 0.1114340422e3)) + 0.2804059680e2 * t24);
    | t17 = t5 * 0.376348799999999983e0;
    | t6 = t9 * t6;
    | t10 = t10 * t4 + t17 + t6;
    | t19 = t18 - t24;
    | t23 = 0.1603245888e1;
    | t2 = t22 * t36 + 0.7790523161e1 * t30 + 0.3504405400e1 * t29 * d4 - 0.7526976000e0 * d4 * (t14 * (-t18 + t24) + t16 * (t18 - t24)) + 0.7464383502e1 * t29 - 0.1318878767e1 * t2 * t28 + t23 * (t14 * t19 - t16 * t19) - 0.2e1 * t27 * (t2 * (t3 * (t16 - t14) - t20) + t21) + t1 * t4 * (t2 * (d4 * t33 + t3 * (0.3010790400e1 * d4 + 0.6412983552e1) + t32) + t3 * t34 + 0.1228085721e2);
    | t4 = 0.1e1 / t15;
    | t14 = t1 * t5;
    | t1 = -t33 * t14 * d4 + t36 * d4 * t31 + t34 * t1 * t9 + t1 * (0.1228085721e2 * t1 + t7 * t3 * (-t38 - 0.1558104632e2)) - t14 * t32 + t26 * t35 + 0.2e1 * t27 * t31 + t31 * t37 + t39 + t40;
    | t3 = t12 - t11;
    | t6 = t6 + t17;
    | Jacob_pinv = [t4 * (t10 * t2 + t13 * t8) t4 * (t1 * t10 + t13 * t2); t4 * (t2 * t6 + t3 * t8) t4 * (t1 * t6 + t3 * t2); t4 * (-t2 * t5 + t8 * t9) t4 * (-t1 * t5 + t2 * t9);];
    | 
    | % Use the pseudoinverse to calculate the desired joint velocities
    | IK_result = Jacob_pinv * [xvel yvel]';
    | 
    | % Write results to outputs, with unit conversion to deg/s and m/s
    | q2vel = IK_result(1) * rad_to_deg;
    | q3vel = IK_result(2) * rad_to_deg;
    | d4vel = IK_result(3);
    | 
    | % Limit output to prevent infinity values
    | if abs(q2vel) > 1000
    |     q2vel = sign(q2vel)*1000;
    | end
    | if abs(q3vel) > 1000
    |     q3vel = sign(q3vel)*1000;
    | end
    | if abs(d4vel) > 10000
    |     d4vel = sign(d4vel)*1000;
    | end
    | % Update result
    | q_vel = [q1vel;q2vel;q3vel;d4vel*100];
    | end
  function loop_control = FK(ref_pos):
    | function loop_control = FK(ref_pos)
    | % This function transforms measured joint positions to the position of the
    | % Tool Center Point. In this case, the TCP is located at the end of the
    | % boom, after the telesopic joint and before the passive joint. After that,
    | % the function checks if TCP position over-pass the collision space so it
    | % will return the suitable control loop
    | %
    | % The first joint angle, q1, has no effect on the kinematics, so it is not
    | % a part of this function.
    | %
    | % Inputs:
    | %   q2,q3,d4    - Current joint positions [deg,m]
    | %
    | % Locals:
    | %   x,y         - Current TCP position position [m]
    | %
    | % Outputs:
    | %   loop_control - suitable control type for reference position
    | %  
    | %
    | 
    | % Modify input joint position
    | q2 = ref_pos(2);
    | q3 = ref_pos(3);
    | d4 = ref_pos(4)/1000;
    | 
    | % Unit conversion to radians and meters
    | deg_to_rad = pi/180;
    | q2 = q2*deg_to_rad;
    | q3 = q3*deg_to_rad;
    | 
    | % Calculate the forward kinematics
    | t1 = cos(q2);
    | t2 = q3 + pi / 0.2e1;
    | t3 = cos(t2);
    | t4 = sin(q2);
    | t2 = sin(t2);
    | t5 = t1 * t2 + t3 * t4;
    | t6 = d4 + 0.213e1;
    | t7 = 0.376348799999999983e0;
    | t8 = 0.350440540000000000e1;
    | t2 = t1 * t3 - t2 * t4;
    | t3 = 0.160450000000000004e1;
    | XY_kin = [t1 * t8 + t5 * t6 + t7 * t2 - ...
    |     0.208160000000000012e0 -t2 * t6 + t4 * t8 + t5 * t7 + t3];
    | 
    | % Write results to outputs (in meters)
    | x = XY_kin(1);
    | y = XY_kin(2);
    | 
    | % Collision limitations
    | x_max = 1.2;
    | y_min = -0.64;
    | 
    | % Check collision limitation over-pass
    | collision = 0;
    | if x < x_max || y < y_min
    |     collision = 1;
    | end
    | 
    | % Generate control type
    | if collision == 1
    |     loop_control = 0;
    | else
    |     loop_control = 1;
    | end
  function ref_position = Move_joints(measurements, ...:
    | function ref_position = Move_joints(measurements, jst_input, ...
    |     Maxi_vel, initial_pos)
    | % This function recieves signals from joystick and calculate new referenced
    | % position.
    | % Parameters and result:
    | %   "measurements": feedback data of the boom position - matrix 4x1
    | %   "jst_input": command signal from joystick - matrix 4x1  
    | %   "Maxi_vel": Maximum velocity of joints - matrix 4x1
    | %   "initial_pos": initial position of the boom when this state is called
    | %   "ref_position": result of this function, which is refernced position of 
    | %                   the boom - matrix 4x1
    | 
    | persistent current_position old_initial
    | step = jst_input .* Maxi_vel;
    | 
    | % If current position is null then set current position is measured data.
    | if isempty(current_position)
    |     current_position = initial_pos;
    |     old_initial = initial_pos;
    | end
    | 
    | % Keep the boom position after changing states
    | if initial_pos ~= old_initial
    |     current_position = initial_pos;
    |     old_initial = initial_pos;    
    | end
    | 
    | if sum(jst_input) ~= 0    
    |     % Update current position with command from joystick       
    |     current_position = measurements + step;        
    | end
    | 
    | % Keep the boom stand still
    | ref_position = current_position;
    | 
    | end
  function ref_position = Move_Tip(measurements, vel_input,...:
    | function ref_position = Move_Tip(measurements, vel_input,...
    |     initial_pos)
    | % This function recieves signals from joystick and calculate new referenced
    | % position as planar movement of the boom.
    | % Parameters and result:
    | %   "measurements": feedback data of the boom position - matrix 4x1
    | %   "vel_input": joints' velocities - matrix 4x1  
    | %   "initial_pos": initial position of the boom when this state is called
    | %   "ref_position": result of this function, which is refernced position of 
    | %                   the boom - matrix 4x1
    | 
    | persistent tcp_position old_initial
    | travel = vel_input;
    | 
    | % If current position is null then set current position is measured data.
    | if isempty(tcp_position)
    |     tcp_position = initial_pos;
    |     old_initial = initial_pos;
    | end
    | 
    | % Keep the boom position after changing states
    | if initial_pos ~= old_initial
    |     tcp_position = initial_pos;
    |     old_initial = initial_pos;    
    | end
    | 
    | % Update current position with command from joystick       
    | if sum(travel) ~= 0 
    |     tcp_position = measurements + travel;        
    | end
    | 
    | % Keep the boom stand still
    | ref_position = tcp_position;
    | 
    | end
  function checked_feedback = checkFeedback(...:
    | function checked_feedback = checkFeedback(measurements, LimitsJoints)
    | % This function checks the referenced positions if they are overpass the 
    | % limits then scales them between the limits.
    | % Parameters and result:
    | %   "measurements": referenced positions - matrix 4x1
    | %   "LimitsJoints": joints' limitations - matrix 4x2  
    | %   "checked_feedback": result of this function, which is referenced 
    | %                       positions of the boom - matrix 4x1
    | 
    |  q1 = measurements(1);
    |  q2 = measurements(2);
    |  q3 = measurements(3);
    |  d4 = measurements(4);
    |  
    |  lim1 = LimitsJoints(1,:);
    |  lim2 = LimitsJoints(2,:);
    |  lim3 = LimitsJoints(3,:);
    |  lim4 = LimitsJoints(4,:);
    |  
    |  % Upper Limits over passed
    |  if q1>lim1(:,2)
    |      q1 = lim1(1,2) - 1;
    |  end
    |  if q2>lim2(:,2)
    |      q2 = lim2(1,2) - 1;
    |  end
    |  if q3>lim3(:,2)
    |      q3 = lim3(1,2) - 1;
    |  end
    |  if d4>lim4(:,2)
    |      d4 = lim4(1,2) - 1;
    |  end
    | 
    | %  Lower Limits over passed
    |  if q1<lim1(:,1)
    |      q1 = lim1(1,1) + 1;
    |  end
    |  if q2<lim2(:,1)
    |      q2 = lim2(1,1) + 1;
    |  end
    |  if q3<lim3(:,1)
    |      q3 = lim3(1,1) + 1;
    |  end
    |  if d4<lim4(:,1)
    |      d4 = lim4(1,1) + 1;
    |  end
    |  % Update result
    |  checked_feedback = [q1; q2; q3; d4];
    |  
    | end
  function checked_input = checkFb_openloop(...:
    | function checked_input = checkFb_openloop(measurements, LimitsJoints,...
    |     jst_input)
    | % This function checks the referenced positions if they are overpass the 
    | % limits then scales them between the limits.
    | % Parameters and result:
    | %   "measurements": referenced positions - matrix 4x1
    | %   "LimitsJoints": joints' limitations - matrix 4x2  
    | %   "checked_feedback": result of this function, which is referenced 
    | %                       positions of the boom - matrix 4x1
    | 
    |  q1 = measurements(1);
    |  q2 = measurements(2);
    |  q3 = measurements(3);
    |  d4 = measurements(4);
    |  
    |  u1 = jst_input(1);
    |  u2 = jst_input(2);
    |  u3 = jst_input(3);
    |  u4 = jst_input(4);
    |  
    |  lim1 = LimitsJoints(1,:);
    |  lim2 = LimitsJoints(2,:);
    |  lim3 = LimitsJoints(3,:);
    |  lim4 = LimitsJoints(4,:);
    |  
    |  % Upper Limits over passed
    |  if q1> (lim1(:,2) - 1)
    |      u1 = 0;
    |  end
    |  if q2> (lim2(:,2) - 1)
    |      u2 = 0;
    |  end
    |  if q3> (lim3(:,2) - 1)
    |      u3 = 0;
    |  end
    |  if d4> (lim4(:,2) - 1)
    |      u4 = 0;
    |  end
    | 
    | %  Lower Limits over passed
    |  if q1< (lim1(:,1) + 1)
    |      u1 = 0;
    |  end
    |  if q2< (lim2(:,1) + 1)
    |      u2 = 0;
    |  end
    |  if q3< (lim3(:,1) + 1)
    |      u3 = 0;
    |  end
    |  if d4< (lim4(:,1) + 1)
    |      u4 = 0;
    |  end
    |  
    |  checked_input = [u1; u2; u3; u4];
    |  
    | end

== matlab function BCS_v1_2018a/Button Input Handler/OpenLoop/Convert ==
  data: y output; u input
function y = fcn(u)
% This function is triggered by joystick button signal. When the function is 
% on, it checks the status of Emergency mode. If Emergency mode is off, it 
% set its status on
% 
% input: 
%     u - status of Emergency mode (1 - on, 0 - off)
% output:
%     y - status of this mode

persistent count

% Set initial status 
if isempty(count)
    count = 0;
end
% Check condition and set suitable status
if u == 0
    if count == 0
        count = 1;
    else
        count = 0;
    end
end
% Return the result
y = count;
end

== matlab function BCS_v1_2018a/Button Input Handler/Tip/Convert ==
  data: y output; u input
function y = fcn(u)
% This function is triggered by joystick button signal. When the function is 
% on, it checks the status of Emergency mode. If Emergency mode is off, it 
% set its status on
% 
% input: 
%     u - status of Emergency mode (1 - on, 0 - off)
% output:
%     y - status of this mode

persistent count

% Set initial status 
if isempty(count)
    count = 0;
end
% Check condition and set suitable status
if u == 0
    if count == 0
        count = 1;
    else
        count = 0;
    end
end
% Return the result
y = count;
end

== matlab function BCS_v1_2018a/Convert to xy coordinates ==
  data: ref_pos input; xy_pos output
function xy_pos = FK_modified(ref_pos)
% This function transforms measured joint positions to the position of the
% Tool Center Point. In this case, the TCP is located at the end of the
% boom, after the telesopic joint and before the passive joint.
%
% The first joint angle, q1, has no effect on the kinematics, so it is not
% a part of this function.
%
% Inputs:
%   ref_pos        - Current joint positions [deg,m] - matrix 4x1
%
% Outputs:
%   xy_pos         - Current TCP position positions [m] - matrix 2x1
%

% Modify input joint position
q2 = ref_pos(2);
q3 = ref_pos(3);
d4 = ref_pos(4)/1000;

% Unit conversion to radians and meters
deg_to_rad = pi/180;
q2 = q2*deg_to_rad;
q3 = q3*deg_to_rad;

% Calculate the forward kinematics
t1 = cos(q2);
t2 = q3 + pi / 0.2e1;
t3 = cos(t2);
t4 = sin(q2);
t2 = sin(t2);
t5 = t1 * t2 + t3 * t4;
t6 = d4 + 0.213e1;
t7 = 0.376348799999999983e0;
t8 = 0.350440540000000000e1;
t2 = t1 * t3 - t2 * t4;
t3 = 0.160450000000000004e1;
XY_kin = [t1 * t8 + t5 * t6 + t7 * t2 - 0.208160000000000012e0 -t2 * t6 + t4 * t8 + t5 * t7 + t3];

% Write results to outputs (in meters)
x = XY_kin(1);
y = XY_kin(2);

xy_pos = [x;y];
end

== matlab function BCS_v1_2018a/Button Input Handler/Joints/Convert ==
  data: y output; u input
function y = fcn(u)
% This function is triggered by joystick button signal. When the function is 
% on, it checks the status of Emergency mode. If Emergency mode is off, it 
% set its status on
% 
% input: 
%     u - status of Emergency mode (1 - on, 0 - off)
% output:
%     y - status of this mode

persistent count

% Set initial status 
if isempty(count)
    count = 0;
end
% Check condition and set suitable status
if u == 0
    if count == 0
        count = 1;
    else
        count = 0;
    end
end
% Return the result
y = count;
end

== matlab function BCS_v1_2018a/Controller/Checking Collision ==
  data: position input; collision output
function collision = boundingbox(position)
% This function checks if input planar position guilds the TCP ovepass the 
% edges of collision area.
% Input:
%     position        - reference position - matrix 2x1
% Output:
%     collision       - Collision status (1 - true, 0 - false)

% Collision edges
x_max = 1.2;
y_min = -0.64;

% Initial value
collision = 0;
% Check collision area overpass
if position(1) < x_max || position(2) < y_min
    collision = 1;
end

end

== matlab function BCS_v1_2018a/Button Input Handler/Emergency/Convert_SoS ==
  data: y output
function y = fcn()
% This function is triggered by joystick button signal to turn on Emergency
% mode
% output:
%     y - status of this mode

persistent count
% Set initial status 
if isempty(count)
    count = 0;
end
% Set suitable status
if count == 0
    count = 1;
else
    count = 0;
end
% Return the result
y = count;
end

== matlab function BCS_v1_2018a/Controller/Convert to xy coordinates ==
  data: ref_pos input; xy_pos output
function xy_pos = FK_modified(ref_pos)
% This function transforms measured joint positions to the position of the
% Tool Center Point. In this case, the TCP is located at the end of the
% boom, after the telesopic joint and before the passive joint.
%
% The first joint angle, q1, has no effect on the kinematics, so it is not
% a part of this function.
%
% Inputs:
%   ref_pos        - Current joint positions [deg,m] - matrix 4x1
%
% Outputs:
%   xy_pos         - Current TCP position positions [m] - matrix 2x1
%

% Modify input joint position
q2 = ref_pos(2);
q3 = ref_pos(3);
d4 = ref_pos(4)/1000;

% Unit conversion to radians and meters
deg_to_rad = pi/180;
q2 = q2*deg_to_rad;
q3 = q3*deg_to_rad;

% Calculate the forward kinematics
t1 = cos(q2);
t2 = q3 + pi / 0.2e1;
t3 = cos(t2);
t4 = sin(q2);
t2 = sin(t2);
t5 = t1 * t2 + t3 * t4;
t6 = d4 + 0.213e1;
t7 = 0.376348799999999983e0;
t8 = 0.350440540000000000e1;
t2 = t1 * t3 - t2 * t4;
t3 = 0.160450000000000004e1;
XY_kin = [t1 * t8 + t5 * t6 + t7 * t2 - 0.208160000000000012e0 -t2 * t6 + t4 * t8 + t5 * t7 + t3];

% Write results to outputs (in meters)
x = XY_kin(1);
y = XY_kin(2);

xy_pos = [x;y];
end
